simulink subsystem "Slip_Control_V2"  (R2026a)
settings: Solver=VariableStepAuto
model mask{Gr=Control.GearRatio, MotorT=Control.MotorTrq, MotorW=Control.MotorW, rwheel=Control.WheelRad, tr=1.24, a=0.871, a_cop=0.8, Af=1.2, P=2350, I=78025, D=11, vx_th=0.7, cd=-2.15, g=9.81, h_CG=0.35, L=1.575, m=320, ro=1.226, Tmax=max(Control.MotorTrq), Load_Ref=[0;400;500;600;700;800;900;1000;1100;1200;1300;1400;1500;1600;1700;1800;1900;2000], Slip_Ref=[0.08;0.08;0.152;0.116;0.102;0.096;0.092;0.09;0.09;0.09;0.094;0.098;0.104;0.112;0.126;0.154;0.232;0.1]}
  mask prompts: Gr "Gear Ratio"; MotorT "Motor Torque"; MotorW "Motor RPM"; rwheel "Wheel Radius"; tr "Rear Track"; a "Front Track to CG"; a_cop "Front Track to CoP"; Af "Frontal Area"; P "Simulink:masks:ProportionalP_MP"; I "Simulink:masks:IntegralI_MP"; D "Simulink:masks:DerivativeD_MP"; vx_th "Activation Velocity"; cd "Lift Coef"; g "Gravitation Acc"; h_CG "CG Height"; L "Wheelbase"; m "Vehcile Mass"; ro "Air Density"; Tmax "Max Torque"; Load_Ref "Reference Load Table"; Slip_Ref "Reference Slip Table"
values from neighbouring files (symbols this model uses):
  rwheel = 0.263    [sm_car_controlparam_SlipControlV2.m]
libraries: slpidlib x2
settings Model: Creator=andrei  LastModifiedBy=andrei

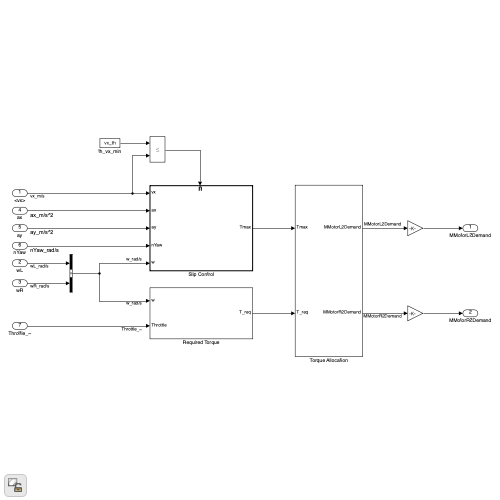
[thumbnail: Simulink's stored preview of the top-level diagram]
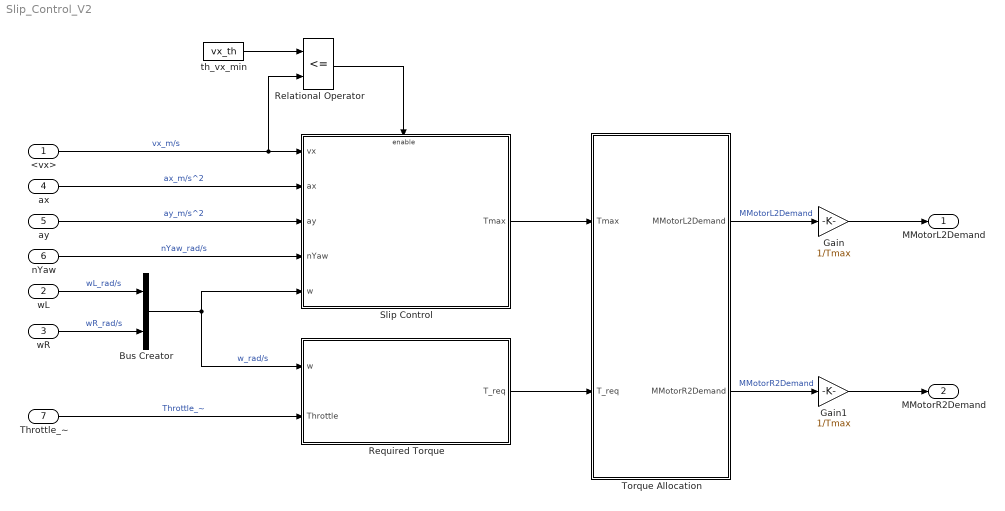
== system Slip_Control_V2 ==
  <vx> : Inport  OutDataTypeStr=double  PortDimensions=1  SampleTime=0
  wL : Inport  Port=2  OutDataTypeStr=double  PortDimensions=1  SampleTime=0
  wR : Inport  Port=3  OutDataTypeStr=double  PortDimensions=1  SampleTime=0
  ax : Inport  Port=4  OutDataTypeStr=double  PortDimensions=1  SampleTime=0
  ay : Inport  Port=5  OutDataTypeStr=double  PortDimensions=1  SampleTime=0
  nYaw : Inport  Port=6  OutDataTypeStr=double  PortDimensions=1  SampleTime=0
  Throttle_~ : Inport  Port=7  OutDataTypeStr=double  PortDimensions=1  SampleTime=0
  Bus Creator : BusCreator  Inputs=2
  Gain : Gain  Gain=1/Tmax
  Gain1 : Gain  Gain=1/Tmax
  Relational Operator : RelationalOperator  Operator=<=  OutDataTypeStr=boolean  RndMeth=Simplest  InputSameDT=off
  Required Torque : Subsystem
  Slip Control : Subsystem
  Torque Allocation : Subsystem
  th_vx_min : Constant  Value=vx_th
  MMotorL2Demand : Outport  OutDataTypeStr=double  PortDimensions=1  SampleTime=0
  MMotorR2Demand : Outport  Port=2  OutDataTypeStr=double  PortDimensions=1  SampleTime=0
  wires:
  Gain1/1 -> MMotorR2Demand/1
  Throttle_~/1 -> Required Torque/2(Throttle)  "Throttle_~"
  Torque Allocation/1(MMotorL2Demand) -> Gain/1  "MMotorL2Demand"
  Required Torque/1(T_req) -> Torque Allocation/2(T_req)
  wL/1 -> Bus Creator/1  "wL_rad/s"
  Bus Creator/1 -> Slip Control/5(w), Required Torque/1(w)  "w_rad/s"
  wR/1 -> Bus Creator/2  "wR_rad/s"
  Torque Allocation/2(MMotorR2Demand) -> Gain1/1  "MMotorR2Demand"
  Gain/1 -> MMotorL2Demand/1
  ax/1 -> Slip Control/2(ax)  "ax_m/s^2"
  ay/1 -> Slip Control/3(ay)  "ay_m/s^2"
  <vx>/1 -> Slip Control/1(vx), Relational Operator/2  "vx_m/s"
  nYaw/1 -> Slip Control/4(nYaw)  "nYaw_rad/s"
  Slip Control/1(Tmax) -> Torque Allocation/1(Tmax)
  Relational Operator/1 -> Slip Control/Enable
  th_vx_min/1 -> Relational Operator/1

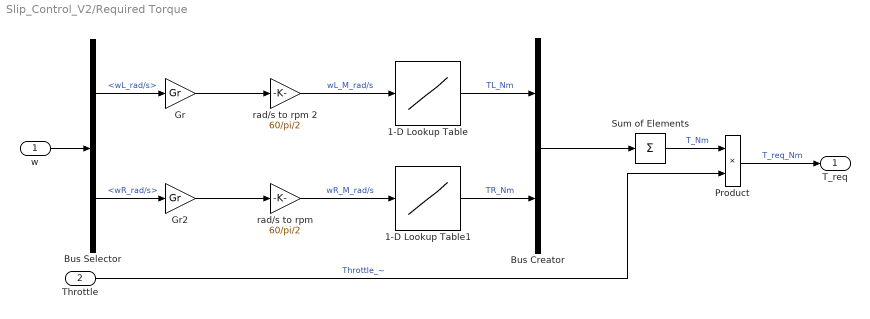
== system Slip_Control_V2/Required Torque ==
  w : Inport
  Throttle : Inport  Port=2
  1-D Lookup Table : Lookup_n-D  NumberOfTableDimensions=1  BreakpointsForDimension1=MotorW  Table=MotorT  InternalRulePriority=Speed  RndMeth=Simplest
  1-D Lookup Table1 : Lookup_n-D  NumberOfTableDimensions=1  BreakpointsForDimension1=MotorW  Table=MotorT  InternalRulePriority=Speed  RndMeth=Simplest
  Bus Creator : BusCreator  Inputs=2
  Bus Selector : BusSelector  OutputSignals=wL_rad/s,wR_rad/s
  Gr : Gain  Gain=Gr
  Gr2 : Gain  Gain=Gr
  Product : Product
  Sum of Elements : Sum  Inputs=+
  rad/s to rpm : Gain  Gain=60/pi/2
  rad/s to rpm 2 : Gain  Gain=60/pi/2
  T_req : Outport
  wires:
  w/1 -> Bus Selector/1
  Sum of Elements/1 -> Product/1  "T_Nm"
  1-D Lookup Table1/1 -> Bus Creator/2  "TR_Nm"
  Throttle/1 -> Product/2  "Throttle_~"
  rad/s to rpm/1 -> 1-D Lookup Table1/1  "wR_M_rad/s"
  Bus Selector/1 -> Gr/1  "<wL_rad/s>"
  Product/1 -> T_req/1  "T_req_Nm"
  Bus Selector/2 -> Gr2/1  "<wR_rad/s>"
  rad/s to rpm 2/1 -> 1-D Lookup Table/1  "wL_M_rad/s"
  1-D Lookup Table/1 -> Bus Creator/1  "TL_Nm"
  Bus Creator/1 -> Sum of Elements/1
  Gr/1 -> rad/s to rpm 2/1
  Gr2/1 -> rad/s to rpm/1

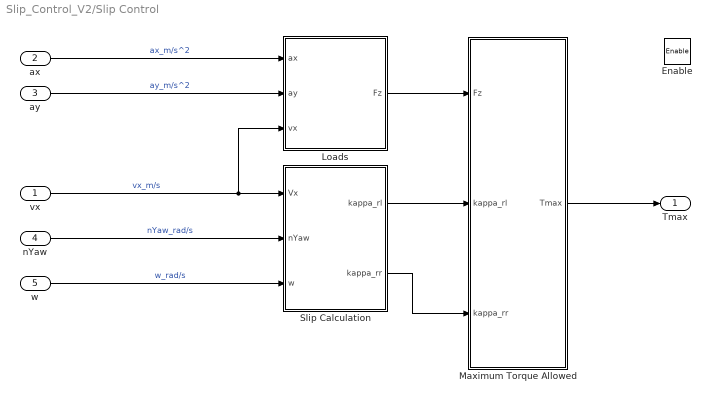
== system Slip_Control_V2/Slip Control ==
  vx : Inport
  ax : Inport  Port=2
  ay : Inport  Port=3
  nYaw : Inport  Port=4
  w : Inport  Port=5
  Enable : EnablePort  StatesWhenEnabling=reset
  Loads : Subsystem
  Maximum Torque Allowed : Subsystem
  Slip Calculation : Subsystem
  Tmax : Outport
  wires:
  Slip Calculation/1(kappa_rl) -> Maximum Torque Allowed/2(kappa_rl)
  Maximum Torque Allowed/1(Tmax) -> Tmax/1
  vx/1 -> Slip Calculation/1(Vx), Loads/3(vx)  "vx_m/s"
  Slip Calculation/2(kappa_rr) -> Maximum Torque Allowed/3(kappa_rr)
  ay/1 -> Loads/2(ay)  "ay_m/s^2"
  Loads/1(Fz) -> Maximum Torque Allowed/1(Fz)
  ax/1 -> Loads/1(ax)  "ax_m/s^2"
  nYaw/1 -> Slip Calculation/2(nYaw)  "nYaw_rad/s"
  w/1 -> Slip Calculation/3(w)  "w_rad/s"

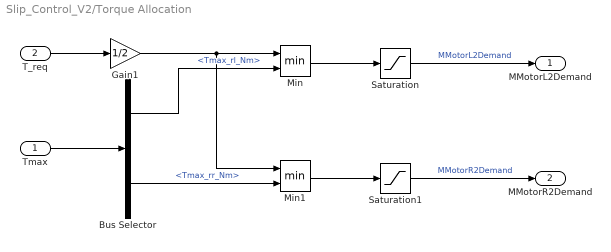
== system Slip_Control_V2/Torque Allocation ==
  Tmax : Inport
  T_req : Inport  Port=2
  Bus Selector : BusSelector  OutputSignals=Tmax_rl_Nm,Tmax_rr_Nm
  Gain1 : Gain  Gain=1/2
  Min : MinMax  Inputs=2
  Min1 : MinMax  Inputs=2
  Saturation : Saturate  UpperLimit=Tmax  LowerLimit=0
  Saturation1 : Saturate  UpperLimit=Tmax  LowerLimit=0
  MMotorL2Demand : Outport
  MMotorR2Demand : Outport  Port=2
  wires:
  Bus Selector/2 -> Min1/2  "<Tmax_rr_Nm>"
  T_req/1 -> Gain1/1
  Gain1/1 -> Min1/1, Min/1
  Min1/1 -> Saturation1/1
  Min/1 -> Saturation/1
  Saturation/1 -> MMotorL2Demand/1  "MMotorL2Demand"
  Saturation1/1 -> MMotorR2Demand/1  "MMotorR2Demand"
  Tmax/1 -> Bus Selector/1
  Bus Selector/1 -> Min/2  "<Tmax_rl_Nm>"

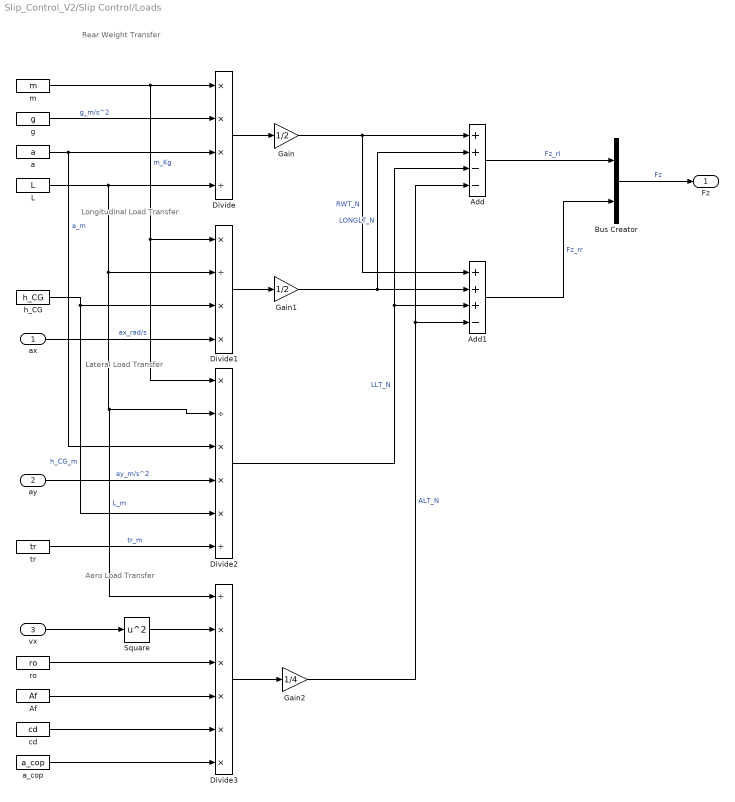
== system Slip_Control_V2/Slip Control/Loads ==
  note: Rear Weight Transfer
  note: Longitudinal Load Transfer
  note: Lateral Load Transfer
  note: Aero Load Transfer
  ax : Inport
  ay : Inport  Port=2
  vx : Inport  Port=3
  Add : Sum  Inputs=++--
  Add1 : Sum  Inputs=+++-
  Af : Constant  Value=Af
  Bus Creator : BusCreator  Inputs=2
  Divide : Product  Inputs=***/
  Divide1 : Product  Inputs=*/**
  Divide2 : Product  Inputs=*/***/
  Divide3 : Product  Inputs=/*****
  Gain : Gain  Gain=1/2
  Gain1 : Gain  Gain=1/2
  Gain2 : Gain  Gain=1/4
  L : Constant  Value=L
  Square : Math  Operator=square
  a : Constant  Value=a
  a_cop : Constant  Value=a_cop
  cd : Constant  Value=cd
  g : Constant  Value=g
  h_CG : Constant  Value=h_CG
  m : Constant  Value=m
  ro : Constant  Value=ro
  tr : Constant  Value=tr
  Fz : Outport
  wires:
  a_cop/1 -> Divide3/6
  cd/1 -> Divide3/5
  Af/1 -> Divide3/4
  ro/1 -> Divide3/3
  Divide3/1 -> Gain2/1
  Bus Creator/1 -> Fz/1  "Fz"
  Add1/1 -> Bus Creator/2  "Fz_rr"
  Add/1 -> Bus Creator/1  "Fz_rl"
  Divide2/1 -> Add1/3, Add/3  "LLT_N"
  tr/1 -> Divide2/6  "tr_m"
  ay/1 -> Divide2/4  "ay_m/s^2"
  Gain1/1 -> Add1/2, Add/2  "LONGLT_N"
  Divide1/1 -> Gain1/1
  ax/1 -> Divide1/4  "ax_rad/s"
  h_CG/1 -> Divide1/3, Divide2/5  "h_CG_m"
  Gain2/1 -> Add1/4, Add/4  "ALT_N"
  Gain/1 -> Add1/1, Add/1  "RWT_N"
  Square/1 -> Divide3/2
  vx/1 -> Square/1
  Divide/1 -> Gain/1
  L/1 -> Divide/4, Divide1/2, Divide2/2, Divide3/1  "L_m"
  a/1 -> Divide2/3, Divide/3  "a_m"
  g/1 -> Divide/2  "g_m/s^2"
  m/1 -> Divide2/1, Divide1/1, Divide/1  "m_Kg"

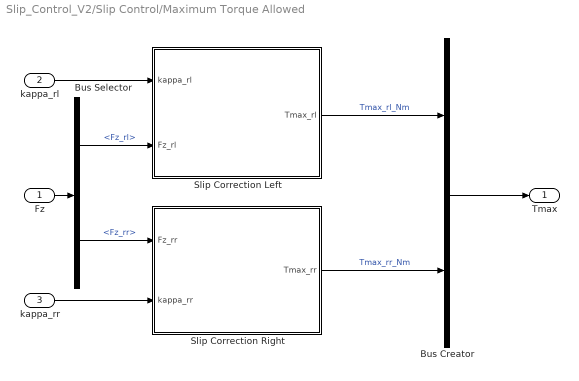
== system Slip_Control_V2/Slip Control/Maximum Torque Allowed ==
  Fz : Inport
  kappa_rl : Inport  Port=2
  kappa_rr : Inport  Port=3
  Bus Creator : BusCreator  Inputs=2
  Bus Selector : BusSelector  OutputSignals=Fz_rl,Fz_rr
  Slip Correction Left : Subsystem
  Slip Correction Right : Subsystem
  Tmax : Outport
  wires:
  Bus Creator/1 -> Tmax/1
  Bus Selector/2 -> Slip Correction Right/1(Fz_rr)  "<Fz_rr>"
  Bus Selector/1 -> Slip Correction Left/2(Fz_rl)  "<Fz_rl>"
  Fz/1 -> Bus Selector/1
  kappa_rr/1 -> Slip Correction Right/2(kappa_rr)
  kappa_rl/1 -> Slip Correction Left/1(kappa_rl)
  Slip Correction Left/1(Tmax_rl) -> Bus Creator/1  "Tmax_rl_Nm"
  Slip Correction Right/1(Tmax_rr) -> Bus Creator/2  "Tmax_rr_Nm"

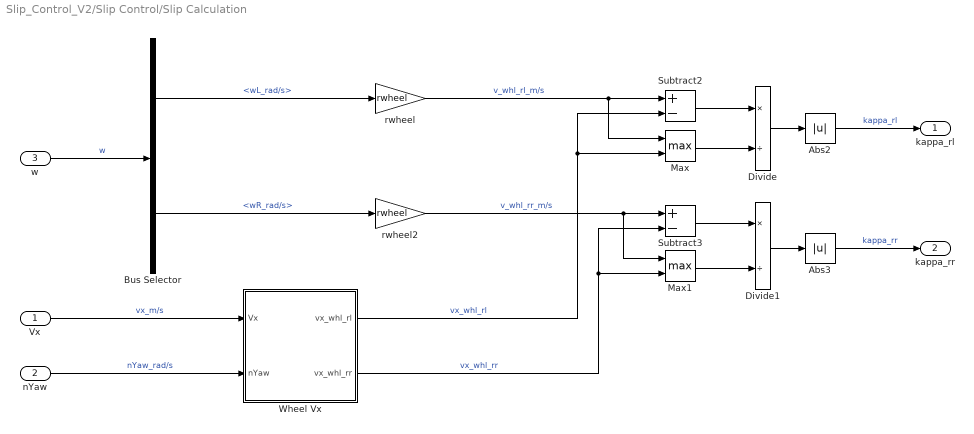
== system Slip_Control_V2/Slip Control/Slip Calculation ==
  Vx : Inport
  nYaw : Inport  Port=2
  w : Inport  Port=3
  Abs2 : Abs  SaturateOnIntegerOverflow=off
  Abs3 : Abs  SaturateOnIntegerOverflow=off
  Bus Selector : BusSelector  OutputSignals=wL_rad/s,wR_rad/s
  Divide : Product  Inputs=*/
  Divide1 : Product  Inputs=*/
  Max : MinMax  Function=max  Inputs=2
  Max1 : MinMax  Function=max  Inputs=2
  Subtract2 : Sum  Inputs=+-
  Subtract3 : Sum  Inputs=+-
  Wheel Vx : Subsystem
  rwheel : Gain  Gain=rwheel
  rwheel2 : Gain  Gain=rwheel
  kappa_rl : Outport
  kappa_rr : Outport  Port=2
  wires:
  Max1/1 -> Divide1/2
  Divide1/1 -> Abs3/1
  Max/1 -> Divide/2
  Divide/1 -> Abs2/1
  Subtract3/1 -> Divide1/1
  Wheel Vx/2(vx_whl_rr) -> Max1/2, Subtract3/2  "vx_whl_rr"
  Subtract2/1 -> Divide/1
  Abs2/1 -> kappa_rl/1  "kappa_rl"
  Wheel Vx/1(vx_whl_rl) -> Max/2, Subtract2/2  "vx_whl_rl"
  Abs3/1 -> kappa_rr/1  "kappa_rr"
  nYaw/1 -> Wheel Vx/2(nYaw)  "nYaw_rad/s"
  rwheel2/1 -> Subtract3/1, Max1/1  "v_whl_rr_m/s"
  rwheel/1 -> Subtract2/1, Max/1  "v_whl_rl_m/s"
  w/1 -> Bus Selector/1  "w"
  Vx/1 -> Wheel Vx/1(Vx)  "vx_m/s"
  Bus Selector/2 -> rwheel2/1  "<wR_rad/s>"
  Bus Selector/1 -> rwheel/1  "<wL_rad/s>"

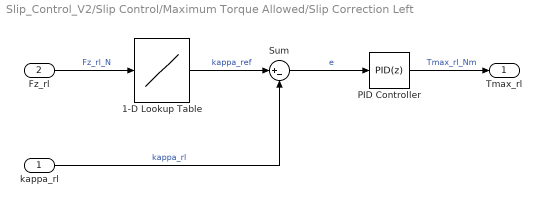
== system Slip_Control_V2/Slip Control/Maximum Torque Allowed/Slip Correction Left ==
  kappa_rl : Inport
  Fz_rl : Inport  Port=2
  1-D Lookup Table : Lookup_n-D  NumberOfTableDimensions=1  BreakpointsForDimension1=Load_Ref  Table=Slip_Ref  ExtrapMethod=Clip  UseLastTableValue=on  InternalRulePriority=Speed  RndMeth=Simplest
  PID Controller : slpidlib/PID Controller  Controller=PID  Form=Parallel  TimeDomain=Discrete-time  UseExternalTs=off  SampleTime=0.005  IntegratorMethod=Forward Euler  FilterMethod=Forward Euler  ControllerParametersSource=internal  P=P  I=I  UseKiTs=off  D=D  UseExternalDerivativeSource=off  N=8  UseFilter=off  TunerSelectOption=Transfer Function Based (PID Tuner App)  InitialConditionSource=internal  InitialConditionForIntegrator=Tmax  InitialConditionForFilter=0  DifferentiatorICPrevScaledInput=Tmax  ExternalReset=none  TrackingMode=off  Kt=1  LimitOutput=on  SatLimitsSource=internal  UpperSaturationLimit=Tmax  LowerSaturationLimit=0  LinearizeAsGain=on  AntiWindupMode=clamping  Kb=1  LimitIntegrator=off  UpperIntegratorSaturationLimit=inf  LowerIntegratorSaturationLimit=-inf  POutMin=[]  POutMax=[]  IOutMin=[]  IOutMax=[]  DOutMin=[]  DOutMax=[]  NOutMin=[]  NOutMax=[]  SumOutMin=[]  SumOutMax=[]  SaturationOutMin=[]  SaturationOutMax=[]  PParamMin=[]  PParamMax=[]  IParamMin=[]  IParamMax=[]  DParamMin=[]  DParamMax=[]  NParamMin=[]  NParamMax=[]  KbParamMin=[]  KbParamMax=[]  KtParamMin=[]  KtParamMax=[]  KbOutMin=[]  KbOutMax=[]  KtOutMin=[]  KtOutMax=[]  IntegratorOutMin=[]  IntegratorOutMax=[]  FilterOutMin=[]  FilterOutMax=[]  SumI1OutMin=[]  SumI1OutMax=[]  SumI2OutMin=[]  SumI2OutMax=[]  SumI3OutMin=[]  SumI3OutMax=[]  SumI4OutMin=[]  SumI4OutMax=[]  SumDOutMin=[]  SumDOutMax=[]  DifferentiatorOutMin=[]  DifferentiatorOutMax=[]  FilterDiffOutCoefMin=[]  FilterDiffOutCoefMax=[]  ReciprocalOutMin=[]  ReciprocalOutMax=[]  SumDenOutMin=[]  SumDenOutMax=[]  SumNumOutMin=[]  SumNumOutMax=[]  DivideOutMin=[]  DivideOutMax=[]  UdiffTsProdOutMin=[]  UdiffTsProdOutMax=[]  NTsProdOutMin=[]  NTsProdOutMax=[]  UintegralTsProdOutMin=[]  UintegralTsProdOutMax=[]  UngainTsProdOutMin=[]  UngainTsProdOutMax=[]  ClampingZeroOutDataTypeStr=Inherit: Inherit via back propagation  ClampingZeroOutMin=[]  ClampingZeroOutMax=[]  FilterDenConstantOutDataTypeStr=Inherit: Inherit via back propagation  FilterDenConstantOutMin=[]  FilterDenConstantOutMax=[]  PCopyOutDataTypeStr=Inherit: Inherit via back propagation  PCopyOutMin=[]  PCopyOutMax=[]  NCopyOutDataTypeStr=Inherit: Inherit via back propagation  NCopyOutMin=[]  NCopyOutMax=[]  IntegratorContinuousStateAttributes=''  IntegratorStateMustResolveToSignalObject=off  IntegratorRTWStateStorageClass=Auto  FilterContinuousStateAttributes=''  FilterStateMustResolveToSignalObject=off  FilterRTWStateStorageClass=Auto  ParallelPVariant=InternalParameters  IdealPVariant=Disabled  IVariant=InternalParameters  DVariant=InternalParameters  IntegratorVariant=Discrete  SatVariant=Enabled  AWVariant=DiscClampingParallel  PCopyVariant=Disabled  TRVariant=Disabled  FdbkBlocksVariant=Forward  IdealPFdbkVariant=Disabled  SatFdbkVariant=Disabled  DerivativeFilterVariant=Differentiator  NVariant=Passthrough  NCopyVariant=Disabled_SignalSpec  FilterICVariant=InternalICsDifferentiator  IntegratorICVariant=InternalICs  ExternalResetVariant=Disabled  TRSumVariant=Passthrough  SumFdbkVariant=Disabled  SumVariant=Sum_PID  TsampFilterVariant=InternalTs  TsampNgainVariant=Passthrough  TsampIntegralVariant=Disabled_SignalSpec  ExternalSaturationOutDataTypeStr=Inherit: Same as second input  DerivativeSourceVariant=ErrorSignal  PreIntVariant=InternalPreInt
  Sum : Sum  Inputs=|+-
  Tmax_rl : Outport
  wires:
  PID Controller/1 -> Tmax_rl/1  "Tmax_rl_Nm"
  Fz_rl/1 -> 1-D Lookup Table/1  "Fz_rl_N"
  Sum/1 -> PID Controller/1  "e"
  1-D Lookup Table/1 -> Sum/1  "kappa_ref"
  kappa_rl/1 -> Sum/2  "kappa_rl"

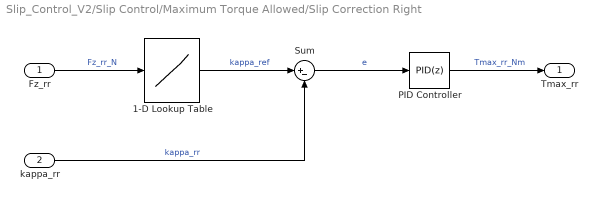
== system Slip_Control_V2/Slip Control/Maximum Torque Allowed/Slip Correction Right ==
  Fz_rr : Inport
  kappa_rr : Inport  Port=2
  1-D Lookup Table : Lookup_n-D  NumberOfTableDimensions=1  BreakpointsForDimension1=Load_Ref  Table=Slip_Ref  ExtrapMethod=Clip  UseLastTableValue=on  InternalRulePriority=Speed  RndMeth=Simplest
  PID Controller : slpidlib/PID Controller  Controller=PID  Form=Parallel  TimeDomain=Discrete-time  UseExternalTs=off  SampleTime=0.005  IntegratorMethod=Forward Euler  FilterMethod=Forward Euler  ControllerParametersSource=internal  P=P  I=I  UseKiTs=off  D=D  UseExternalDerivativeSource=off  N=8  UseFilter=off  TunerSelectOption=Transfer Function Based (PID Tuner App)  InitialConditionSource=internal  InitialConditionForIntegrator=Tmax  InitialConditionForFilter=0  DifferentiatorICPrevScaledInput=Tmax  ExternalReset=none  TrackingMode=off  Kt=1  LimitOutput=on  SatLimitsSource=internal  UpperSaturationLimit=Tmax  LowerSaturationLimit=0  LinearizeAsGain=on  AntiWindupMode=clamping  Kb=1  LimitIntegrator=off  UpperIntegratorSaturationLimit=inf  LowerIntegratorSaturationLimit=-inf  POutMin=[]  POutMax=[]  IOutMin=[]  IOutMax=[]  DOutMin=[]  DOutMax=[]  NOutMin=[]  NOutMax=[]  SumOutMin=[]  SumOutMax=[]  SaturationOutMin=[]  SaturationOutMax=[]  PParamMin=[]  PParamMax=[]  IParamMin=[]  IParamMax=[]  DParamMin=[]  DParamMax=[]  NParamMin=[]  NParamMax=[]  KbParamMin=[]  KbParamMax=[]  KtParamMin=[]  KtParamMax=[]  KbOutMin=[]  KbOutMax=[]  KtOutMin=[]  KtOutMax=[]  IntegratorOutMin=[]  IntegratorOutMax=[]  FilterOutMin=[]  FilterOutMax=[]  SumI1OutMin=[]  SumI1OutMax=[]  SumI2OutMin=[]  SumI2OutMax=[]  SumI3OutMin=[]  SumI3OutMax=[]  SumI4OutMin=[]  SumI4OutMax=[]  SumDOutMin=[]  SumDOutMax=[]  DifferentiatorOutMin=[]  DifferentiatorOutMax=[]  FilterDiffOutCoefMin=[]  FilterDiffOutCoefMax=[]  ReciprocalOutMin=[]  ReciprocalOutMax=[]  SumDenOutMin=[]  SumDenOutMax=[]  SumNumOutMin=[]  SumNumOutMax=[]  DivideOutMin=[]  DivideOutMax=[]  UdiffTsProdOutMin=[]  UdiffTsProdOutMax=[]  NTsProdOutMin=[]  NTsProdOutMax=[]  UintegralTsProdOutMin=[]  UintegralTsProdOutMax=[]  UngainTsProdOutMin=[]  UngainTsProdOutMax=[]  ClampingZeroOutDataTypeStr=Inherit: Inherit via back propagation  ClampingZeroOutMin=[]  ClampingZeroOutMax=[]  FilterDenConstantOutDataTypeStr=Inherit: Inherit via back propagation  FilterDenConstantOutMin=[]  FilterDenConstantOutMax=[]  PCopyOutDataTypeStr=Inherit: Inherit via back propagation  PCopyOutMin=[]  PCopyOutMax=[]  NCopyOutDataTypeStr=Inherit: Inherit via back propagation  NCopyOutMin=[]  NCopyOutMax=[]  IntegratorContinuousStateAttributes=''  IntegratorStateMustResolveToSignalObject=off  IntegratorRTWStateStorageClass=Auto  FilterContinuousStateAttributes=''  FilterStateMustResolveToSignalObject=off  FilterRTWStateStorageClass=Auto  ParallelPVariant=InternalParameters  IdealPVariant=Disabled  IVariant=InternalParameters  DVariant=InternalParameters  IntegratorVariant=Discrete  SatVariant=Enabled  AWVariant=DiscClampingParallel  PCopyVariant=Disabled  TRVariant=Disabled  FdbkBlocksVariant=Forward  IdealPFdbkVariant=Disabled  SatFdbkVariant=Disabled  DerivativeFilterVariant=Differentiator  NVariant=Passthrough  NCopyVariant=Disabled_SignalSpec  FilterICVariant=InternalICsDifferentiator  IntegratorICVariant=InternalICs  ExternalResetVariant=Disabled  TRSumVariant=Passthrough  SumFdbkVariant=Disabled  SumVariant=Sum_PID  TsampFilterVariant=InternalTs  TsampNgainVariant=Passthrough  TsampIntegralVariant=Disabled_SignalSpec  ExternalSaturationOutDataTypeStr=Inherit: Same as second input  DerivativeSourceVariant=ErrorSignal  PreIntVariant=InternalPreInt
  Sum : Sum  Inputs=|+-
  Tmax_rr : Outport
  wires:
  PID Controller/1 -> Tmax_rr/1  "Tmax_rr_Nm"
  Sum/1 -> PID Controller/1  "e"
  kappa_rr/1 -> Sum/2  "kappa_rr"
  1-D Lookup Table/1 -> Sum/1  "kappa_ref"
  Fz_rr/1 -> 1-D Lookup Table/1  "Fz_rr_N"

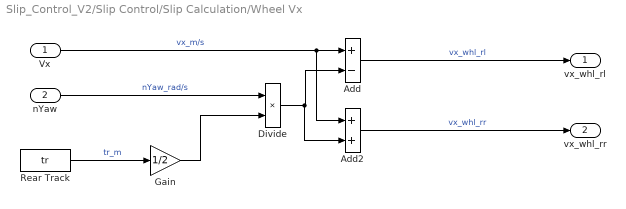
== system Slip_Control_V2/Slip Control/Slip Calculation/Wheel Vx ==
  Vx : Inport
  nYaw : Inport  Port=2
  Add : Sum  Inputs=+-
  Add2 : Sum
  Divide : Product  Inputs=**
  Gain : Gain  Gain=1/2
  Rear Track : Constant  Value=tr
  vx_whl_rl : Outport
  vx_whl_rr : Outport  Port=2
  wires:
  Add2/1 -> vx_whl_rr/1  "vx_whl_rr"
  Add/1 -> vx_whl_rl/1  "vx_whl_rl"
  Divide/1 -> Add/2, Add2/2
  Vx/1 -> Add/1, Add2/1  "vx_m/s"
  Gain/1 -> Divide/2
  nYaw/1 -> Divide/1  "nYaw_rad/s"
  Rear Track/1 -> Gain/1  "tr_m"
